simulink model "Sawyer_simulink_model"  (R2017a)
settings: Solver=FixedStepAuto  StartTime=0.0  StopTime=tf  FixedStep=maxstep  MaxStep=maxstep  RelTol=tol  AbsTol=tol  EnableMultiTasking=on
values from neighbouring files (symbols this model uses):
  ctltyp = 0    [two_dof_sim.m]
  damping_coeffs = diag([0 0])    [two_dof_sim.m]
  Kd = diag([1 3])    [two_dof_sim.m]
  Kp = diag([3 10])    [two_dof_sim.m]
  theta0 = [0;pi/2]    [two_dof_sim.m]
  thetadot0 = [0;0]    [two_dof_sim.m]
  thset = [1;pi/2+0.5]    [two_dof_sim.m]
  type = 1    [two_dof_sim.m]
settings Model: Creator=winckrc  LastModifiedBy=localmgr
settings DataIOCC: LimitDataPoints=on  SaveFormat=Array
settings OptimizationCC: LifeSpan=inf
settings DebuggingCC: SFUnexpectedBacktrackingDiag=warning  SFNoUnconditionalDefaultTransitionDiag=warning  SFExecutionAtInitializationDiag=none
settings HardwareCC: ProdBitPerPointer=32  ProdBitPerSizeT=32  ProdBitPerPtrDiffT=32  ProdLargestAtomicFloat=None  ProdIntDivRoundTo=Undefined  ProdEndianess=Unspecified  ProdWordSize=32  ProdHWDeviceType=32-bit Generic
settings ModelReferenceCC: PropagateSignalLabelsOutOfModel=off
settings GRTTargetCC: TargetLangStandard=C89/C90 (ANSI)  GeneratePreprocessorConditionals=Disable all
settings ConfigComp: CovMetricSettings=dw  CovHtmlReporting=on  CovSaveCumulativeToWorkspaceVar=on  CovSaveSingleToWorkspaceVar=on  CovExternalEMLEnable=off

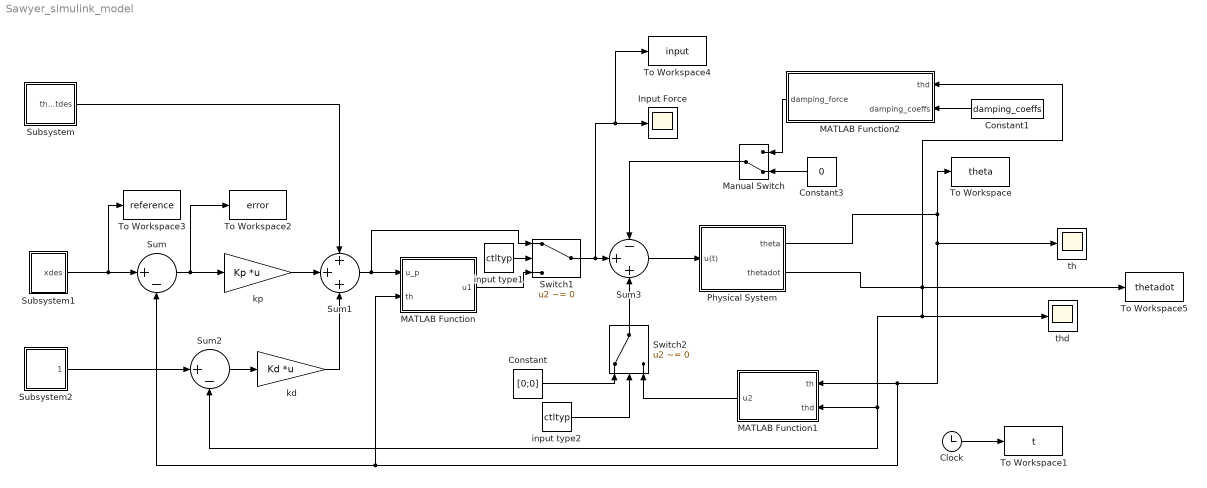
== system Sawyer_simulink_model ==
  Clock : Clock
  Constant : Constant  Value=[0;0]
  Constant1 : Constant  Value=damping_coeffs
  Constant3 : Constant  Value=0
  Input Force : Scope
  MATLAB Function : MATLAB Function  TreatAsAtomicUnit=on
  MATLAB Function1 : MATLAB Function  TreatAsAtomicUnit=on
  MATLAB Function2 : MATLAB Function  TreatAsAtomicUnit=on
  Manual Switch : ManualSwitch  CurrentSetting=0
  Physical System : Subsystem
  Subsystem : Subsystem
  Subsystem1 : Subsystem
  Subsystem2 : Subsystem
  Sum : Sum  Inputs=|+-
  Sum1 : Sum  Inputs=+++
  Sum2 : Sum  Inputs=|+-
  Sum3 : Sum  Inputs=-++
  Switch1 : Switch  Criteria=u2 ~= 0  Threshold=1.5
  Switch2 : Switch  Criteria=u2 ~= 0  Threshold=1.5
  To Workspace : ToWorkspace  VariableName=theta  SampleTime=-1
  To Workspace1 : ToWorkspace  VariableName=t  SampleTime=-1
  To Workspace2 : ToWorkspace  VariableName=error  SampleTime=-1
  To Workspace3 : ToWorkspace  VariableName=reference  SampleTime=-1
  To Workspace4 : ToWorkspace  VariableName=input  SampleTime=-1
  To Workspace5 : ToWorkspace  VariableName=thetadot  SampleTime=-1
  input type1 : Constant  Value=ctltyp
  input type2 : Constant  Value=ctltyp
  kd : Gain  Gain=Kd  Multiplication=Matrix(K*u) (u vector)
  kp : Gain  Gain=Kp  Multiplication=Matrix(K*u) (u vector)
  th : Scope
  thd : Scope
  wires:
  Clock/1 -> To Workspace1/1
  MATLAB Function2/1(damping_force) -> Manual Switch/1
  Constant3/1 -> Manual Switch/2
  Manual Switch/1 -> Sum3/1
  kd/1 -> Sum1/3
  Sum2/1 -> kd/1
  Subsystem2/1(xdotdes) -> Sum2/1
  kp/1 -> Sum1/2
  Subsystem1/1(xdes) -> Sum/1, To Workspace3/1
  Subsystem/1(thddotdes) -> Sum1/1
  Sum/1 -> To Workspace2/1, kp/1
  Switch1/1 -> Input Force/1, To Workspace4/1, Sum3/2
  Sum1/1 -> Switch1/1, MATLAB Function/1(u_p)
  input type1/1 -> Switch1/2
  MATLAB Function/1(u1) -> Switch1/3
  input type2/1 -> Switch2/2
  Constant/1 -> Switch2/1
  MATLAB Function1/1(u2) -> Switch2/3
  Switch2/1 -> Sum3/3
  Constant1/1 -> MATLAB Function2/2(damping_coeffs)
  Sum3/1 -> Physical System/1(u(t))
  Physical System/2(thetadot) -> To Workspace5/1, MATLAB Function1/2(thd), Sum2/2, thd/1, MATLAB Function2/1(thd)
  Physical System/1(theta) -> MATLAB Function1/1(th), MATLAB Function/2(th), Sum/2, th/1, To Workspace/1

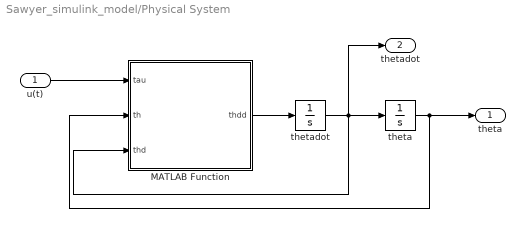
== system Sawyer_simulink_model/Physical System ==
  u(t) : Inport
  MATLAB Function : MATLAB Function  TreatAsAtomicUnit=on
  "theta " : Integrator  InitialCondition=theta0
  "thetadot " : Integrator  InitialCondition=thetadot0
  theta : Outport
  thetadot : Outport  Port=2
  wires:
  "thetadot "/1 -> thetadot/1, MATLAB Function/3(thd), "theta "/1
  MATLAB Function/1(thdd) -> "thetadot "/1
  u(t)/1 -> MATLAB Function/1(tau)
  "theta "/1 -> theta/1, MATLAB Function/2(th)

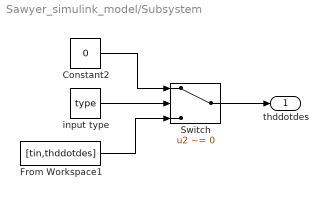
== system Sawyer_simulink_model/Subsystem ==
  Constant2 : Constant  Value=0
  From Workspace1 : FromWorkspace  VariableName=[tin,thddotdes]  SampleTime=0  OutputAfterFinalValue=Setting to zero
  Switch : Switch  Criteria=u2 ~= 0  Threshold=1.5
  input type : Constant  Value=type
  thddotdes : Outport
  wires:
  Constant2/1 -> Switch/1
  From Workspace1/1 -> Switch/3
  input type/1 -> Switch/2
  Switch/1 -> thddotdes/1

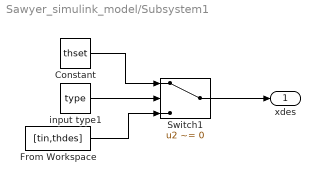
== system Sawyer_simulink_model/Subsystem1 ==
  Constant : Constant  Value=thset
  From Workspace : FromWorkspace  VariableName=[tin,thdes]  SampleTime=0  OutputAfterFinalValue=Holding final value
  Switch1 : Switch  Criteria=u2 ~= 0  Threshold=1.5
  input type1 : Constant  Value=type
  xdes : Outport
  wires:
  input type1/1 -> Switch1/2
  Constant/1 -> Switch1/1
  Switch1/1 -> xdes/1
  From Workspace/1 -> Switch1/3

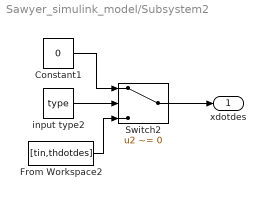
== system Sawyer_simulink_model/Subsystem2 ==
  Constant1 : Constant  Value=0
  From Workspace2 : FromWorkspace  VariableName=[tin,thdotdes]  SampleTime=0  OutputAfterFinalValue=Setting to zero
  Switch2 : Switch  Criteria=u2 ~= 0  Threshold=1.5
  input type2 : Constant  Value=type
  xdotdes : Outport
  wires:
  input type2/1 -> Switch2/2
  Constant1/1 -> Switch2/1
  Switch2/1 -> xdotdes/1
  From Workspace2/1 -> Switch2/3

== matlab function Sawyer_simulink_model/MATLAB Function ==
  data: u_p input; th input; u1 output
function u1  = fcn(u_p,th)

Mhat = M_func(th(1),th(2));

% Mhat = eye(2);

 u1 = Mhat*u_p;

== matlab function Sawyer_simulink_model/Physical System/MATLAB Function ==
  data: tau input; th input; thdd output; thd input
function thdd  = fcn(tau,th,thd)

M = M_func(th(1),th(2));
G = G_func(th(1),th(2));
C = C_func(th(1),th(2));
B = B_func(th(1),th(2));

thdd = M\( tau - C*(thd.^2) - B*thdthdfunc(thd) - G);

== matlab function Sawyer_simulink_model/MATLAB Function1 ==
  data: th input; u2 output; thd input
function u2 = fcn(th,thd)

G = G_func(th(1),th(2));
C = C_func(th(1),th(2));
B = B_func(th(1),th(2));

u2 = C*thd.^2 + B*thdthdfunc(thd) + G;

== matlab function Sawyer_simulink_model/MATLAB Function2 ==
  data: thd input; damping_force output; damping_coeffs input
function damping_force = fcn(thd,damping_coeffs)
damping_force = damping_coeffs*thd;
